simulink model "SC_FFNN_trainlm_15_15_15_15_Dec_8"  (R2021a)
settings: Solver=VariableStepAuto  StartTime=0.0  StopTime=T  FixedStep=0.1  MaxStep=.1  RelTol=1e-3
model workspace (MAT data in the model file):
  T = [0 0.05 0.1 0.15 0.2 0.25 0.3 0.35 0.4 0.45 0.5 0.55 ... (701 elements, 701x1)]
  U = [3.99594136536 3.99594136536 3.99594136536 3.99594136536 3.99594136536 3.99594136536 3.99594136536 3.99594136536 3.99594136536 3.99594136536 3.99594136536 3.99594136536 ... (701 elements, 701x1)]
libraries: neural x66, simulink_extras x2
(part 2 of 3)

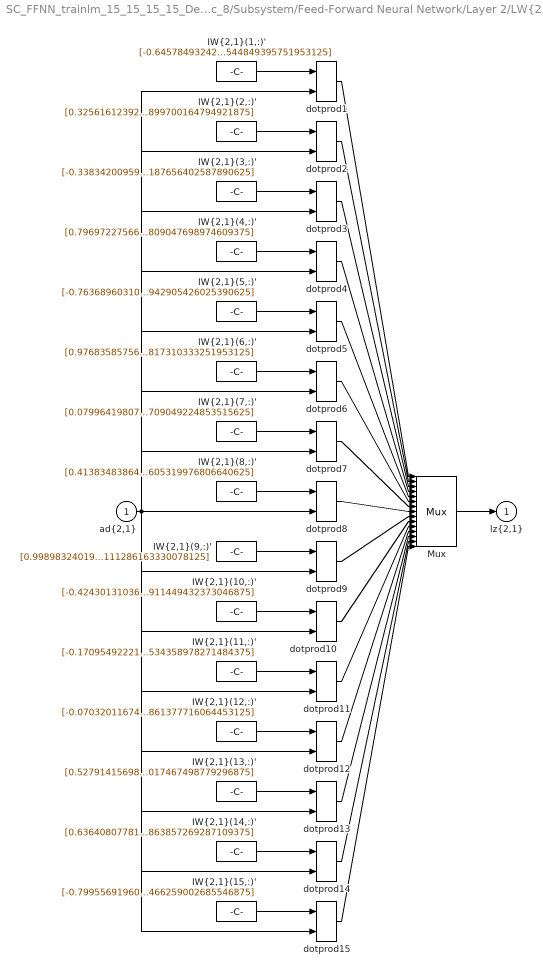
== system SC_FFNN_trainlm_15_15_15_15_Dec_8/Subsystem/Feed-Forward Neural Network/Layer 2/LW{2,1} ==
  "ad{2,1}" : Inport  PortDimensions=15
      mask Display: e = 0.06;c1 = [120 230 180]/255;c2 = ([120 230 180]+0)/(256+128);c3 = ([120 230 180]+128)/(256+128);patch([0 1 1 0],[0 0 1 1],c1);patch([0 1 1 1-e 1-e 0+e],[0 0 1 1-e 0+e 0+e],c2);patch([0 0 1 1-e 0+e 0+e],[0 1 1 1-e 1-e 0+e],c3);plot([0 1 1 0 0],[0 0 1 1 0]);
  "IW{2,1}(1,:)'" : Constant  Value=[-0.6457849324217816988635831876308657228946685791015625;-0.643766092226467190329231016221456229686737060546875;-0.63161180496894697711240951321087777614593505859375;-0.0878846663125170124430951545946300029754638671875;0.0675439035340004156893201070488430559635162353515625;0.3850639727730376105085952076478861272335052490234375;-0.897336227775257899708094555535353720188140869140625;0.4800646559755552544856982422061264514923095703125;-0.5886509570704803184781894742627628147602081298828125;-0.7754320756879466980393544872640632092952728271484375;-0.0247924491321527273868241536547429859638214111328125;-0.81529532256159686909313677460886538028717041015625;-0.367142001707418064171406513196416199207305908203125;0.9758694699049907939070180873386561870574951171875;-0.2984465102282147785928145822254009544849395751953125]
      mask Display: e = 0.06;c1 = [120 150 230]/255;c2 = ([120 150 230]+0)/383;c3 = ([120 150 230]+128)/383;patch([0 1 1 0],[0 0 1 1],c1);patch([0 1 1 1-e 1-e 0+e],[0 0 1 1-e 0+e 0+e],c2);patch([0 0 1 1-e 0+e 0+e],[0 1 1 1-e 1-e 0+e],c3);plot([0 1 1 0 0],[0 0 1 1 0]);disp('weights');
  "IW{2,1}(10,:)'" : Constant  Value=[-0.4243013103697255150592582140234299004077911376953125;-0.0630636001920052979841102569480426609516143798828125;-0.261951995923644875841063139887410216033458709716796875;0.583812871633243357649689642130397260189056396484375;0.2295210394552672783508029397125937975943088531494140625;-0.76428735103558020913538939566933549940586090087890625;-0.553496390046050112943021304090507328510284423828125;0.2202211617163360724003240420643123798072338104248046875;-0.398874395379135215922161705748294480144977569580078125;0.32329322708284891074725919679622165858745574951171875;-0.69601770115887873213722514265100471675395965576171875;-0.76362015015753226254702212827396579086780548095703125;0.8276008215591357242146841599605977535247802734375;0.364025398305722613923052222162368707358837127685546875;-0.1547086935590751277658227991196326911449432373046875]
      mask Display: e = 0.06;c1 = [120 150 230]/255;c2 = ([120 150 230]+0)/383;c3 = ([120 150 230]+128)/383;patch([0 1 1 0],[0 0 1 1],c1);patch([0 1 1 1-e 1-e 0+e],[0 0 1 1-e 0+e 0+e],c2);patch([0 0 1 1-e 0+e 0+e],[0 1 1 1-e 1-e 0+e],c3);plot([0 1 1 0 0],[0 0 1 1 0]);disp('weights');
  "IW{2,1}(11,:)'" : Constant  Value=[-0.170954922213783166995426654466427862644195556640625;0.82426494847924569597807931131683290004730224609375;-0.97343359906549498106187456869520246982574462890625;0.262139998427187048690711890230886638164520263671875;0.0522049315911223832387122456566430628299713134765625;0.0990802140303959077982653980143368244171142578125;0.2814358459318511140878626974881626665592193603515625;0.5787278872838108600973328066174872219562530517578125;-0.5252539605888415508161415345966815948486328125;-0.780489898553896832567033925442956387996673583984375;-0.3683771233222679075680616733734495937824249267578125;-0.8028118145780045455950357791152782738208770751953125;0.4134304353938611509278189259930513799190521240234375;-0.691260389041455258762880475842393934726715087890625;-0.2807873640555287320097477277158759534358978271484375]
      mask Display: e = 0.06;c1 = [120 150 230]/255;c2 = ([120 150 230]+0)/383;c3 = ([120 150 230]+128)/383;patch([0 1 1 0],[0 0 1 1],c1);patch([0 1 1 1-e 1-e 0+e],[0 0 1 1-e 0+e 0+e],c2);patch([0 0 1 1-e 0+e 0+e],[0 1 1 1-e 1-e 0+e],c3);plot([0 1 1 0 0],[0 0 1 1 0]);disp('weights');
  "IW{2,1}(12,:)'" : Constant  Value=[-0.0703201167497253809557378190220333635807037353515625;-0.7919768504412429965810815701843239367008209228515625;0.06419107271674366621549978617622400633990764617919921875;-0.317608463431375775964937702156021259725093841552734375;0.7925487488476712361062936906819231808185577392578125;0.00801786996665575062148700880015894654206931591033935546875;-0.047812738308209347393162857997594983316957950592041015625;0.029586733863963689261655787277049967087805271148681640625;0.345442257577304456805933341456693597137928009033203125;1.329969655156431063147692839265801012516021728515625;1.0607839833820345010195751456194557249546051025390625;-0.3838467293922487311164104539784602820873260498046875;0.1155779335097524285203007821110077202320098876953125;-0.32214951211426579025243199794203974306583404541015625;0.116638399738594245036438223905861377716064453125]
      mask Display: e = 0.06;c1 = [120 150 230]/255;c2 = ([120 150 230]+0)/383;c3 = ([120 150 230]+128)/383;patch([0 1 1 0],[0 0 1 1],c1);patch([0 1 1 1-e 1-e 0+e],[0 0 1 1-e 0+e 0+e],c2);patch([0 0 1 1-e 0+e 0+e],[0 1 1 1-e 1-e 0+e],c3);plot([0 1 1 0 0],[0 0 1 1 0]);disp('weights');
  "IW{2,1}(13,:)'" : Constant  Value=[0.5279141569839131964414491449133493006229400634765625;0.4910921474034346534409678497468121349811553955078125;-0.606683617264736074758957329322583973407745361328125;-0.8382751537393726692926065879873931407928466796875;0.414506970630843074587801311281509697437286376953125;0.7809513583688765248069785229745320975780487060546875;0.3076240451915472906563309152261354029178619384765625;-0.5879442809896107124956188272335566580295562744140625;-0.81700253732117555927061403053812682628631591796875;-0.62507838715662700224129366688430309295654296875;0.3928659780121896982763018968398682773113250732421875;-0.6634974030169444869642347839544527232646942138671875;-0.3731420201268174086095541497343219816684722900390625;-0.6777320563012783072309730414417572319507598876953125;0.4850907314038781503739983236300759017467498779296875]
      mask Display: e = 0.06;c1 = [120 150 230]/255;c2 = ([120 150 230]+0)/383;c3 = ([120 150 230]+128)/383;patch([0 1 1 0],[0 0 1 1],c1);patch([0 1 1 1-e 1-e 0+e],[0 0 1 1-e 0+e 0+e],c2);patch([0 0 1 1-e 0+e 0+e],[0 1 1 1-e 1-e 0+e],c3);plot([0 1 1 0 0],[0 0 1 1 0]);disp('weights');
  "IW{2,1}(14,:)'" : Constant  Value=[0.636408077815341588490127833210863173007965087890625;0.4725349111932770629351807656348682940006256103515625;-0.8132589664898139947268873584107495844364166259765625;0.554481073097886412170964831602759659290313720703125;0.5627541035985543782516060673515312373638153076171875;0.597920557625758686270955877262167632579803466796875;0.498262926207038159276407895958982408046722412109375;-0.8266669052089354874368609671364538371562957763671875;-0.189369160238817446639814079389907419681549072265625;-0.4676423221847223476999033664469607174396514892578125;-0.7493356377816400293312426583725027740001678466796875;-0.6075021554860893235883168017608113586902618408203125;-0.6675928741956986822714270601863972842693328857421875;0.516224862654837135522711832891218364238739013671875;-0.1513304327486186817708357921219430863857269287109375]
      mask Display: e = 0.06;c1 = [120 150 230]/255;c2 = ([120 150 230]+0)/383;c3 = ([120 150 230]+128)/383;patch([0 1 1 0],[0 0 1 1],c1);patch([0 1 1 1-e 1-e 0+e],[0 0 1 1-e 0+e 0+e],c2);patch([0 0 1 1-e 0+e 0+e],[0 1 1 1-e 1-e 0+e],c3);plot([0 1 1 0 0],[0 0 1 1 0]);disp('weights');
  "IW{2,1}(15,:)'" : Constant  Value=[-0.799556919609016869543438588152639567852020263671875;0.12372285056327481100879595032893121242523193359375;-0.3508058136455447506563132265000604093074798583984375;0.982529142477143846434728402527980506420135498046875;-0.2530487716218956517622018509428016841411590576171875;0.44291456538828744005087401092168875038623809814453125;0.499890054502398040181532223868998698890209197998046875;0.56521538701470941390425650752149522304534912109375;-0.71049396982996892990769310927134938538074493408203125;0.44869860757813551099815185807528905570507049560546875;-0.64834895004813952734679105560644529759883880615234375;-0.50962148200618540005990553254378028213977813720703125;0.244994518559790375178408794454298913478851318359375;0.99033985712147754032486091091413982212543487548828125;-0.1412884228475899117682956784847192466259002685546875]
      mask Display: e = 0.06;c1 = [120 150 230]/255;c2 = ([120 150 230]+0)/383;c3 = ([120 150 230]+128)/383;patch([0 1 1 0],[0 0 1 1],c1);patch([0 1 1 1-e 1-e 0+e],[0 0 1 1-e 0+e 0+e],c2);patch([0 0 1 1-e 0+e 0+e],[0 1 1 1-e 1-e 0+e],c3);plot([0 1 1 0 0],[0 0 1 1 0]);disp('weights');
  "IW{2,1}(2,:)'" : Constant  Value=[0.325616123921948830144401654251851141452789306640625;-0.2807301730358393587749787911889143288135528564453125;0.19442270067570976976867314078845083713531494140625;-0.7966612127504897333807321047061122953891754150390625;-0.7816915759150828701962154809734784066677093505859375;0.1133396699280251329611246546846814453601837158203125;-0.854229401802047760838831891305744647979736328125;-0.530346170504191416483763532596640288829803466796875;-0.2234567379043965740237354111741296947002410888671875;0.5688557814878254514923128226655535399913787841796875;0.5379165281177382684774102017399854958057403564453125;-0.9843594128613302185470956828794442117214202880859375;-0.564873381154358700229067835607565939426422119140625;-0.6591359538862333611319854753674007952213287353515625;0.3710714174950744403957969552720896899700164794921875]
      mask Display: e = 0.06;c1 = [120 150 230]/255;c2 = ([120 150 230]+0)/383;c3 = ([120 150 230]+128)/383;patch([0 1 1 0],[0 0 1 1],c1);patch([0 1 1 1-e 1-e 0+e],[0 0 1 1-e 0+e 0+e],c2);patch([0 0 1 1-e 0+e 0+e],[0 1 1 1-e 1-e 0+e],c3);plot([0 1 1 0 0],[0 0 1 1 0]);disp('weights');
  "IW{2,1}(3,:)'" : Constant  Value=[-0.33834200959339089109789711073972284793853759765625;-0.8865906218634176383375233854167163372039794921875;-0.4001260198204221740780894833733327686786651611328125;1.02120211881773759188263284158892929553985595703125;0.70838934016579579999728366601630114018917083740234375;-0.1764984869556638358290001633577048778533935546875;-0.8229450806505591575756852762424387037754058837890625;0.52977589563979499143187013032729737460613250732421875;0.184675824070698435530601955179008655250072479248046875;-0.329453926740678137985440798729541711509227752685546875;-0.1473086768571251481407813344048918224871158599853515625;-0.1490037611855022092743894290833850391209125518798828125;-0.4979163079685278159303152278880588710308074951171875;-0.4844154988559739027920159060158766806125640869140625;-0.4117027324643007801796557032503187656402587890625]
      mask Display: e = 0.06;c1 = [120 150 230]/255;c2 = ([120 150 230]+0)/383;c3 = ([120 150 230]+128)/383;patch([0 1 1 0],[0 0 1 1],c1);patch([0 1 1 1-e 1-e 0+e],[0 0 1 1-e 0+e 0+e],c2);patch([0 0 1 1-e 0+e 0+e],[0 1 1 1-e 1-e 0+e],c3);plot([0 1 1 0 0],[0 0 1 1 0]);disp('weights');
  "IW{2,1}(4,:)'" : Constant  Value=[0.7969722756685990727731905280961655080318450927734375;0.0437713473225584959180878286133520305156707763671875;-0.5997826501763905415742783588939346373081207275390625;-0.253376872142529852016679114967701025307178497314453125;-0.253880698516011638066203204289195127785205841064453125;-0.8411563306374827408973260389757342636585235595703125;0.5967017282279047929449689036118797957897186279296875;0.901428807425623812576986892963759601116180419921875;-0.4921638283901297317157741417759098112583160400390625;0.14982480718348611947732251792331226170063018798828125;-0.48965927940785081151631175089278258383274078369140625;0.300741058062357069502468220889568328857421875;0.785844810571953988898030729615129530429840087890625;-0.2064013627337126788319210390909574925899505615234375;0.0612586077137711182416524025029502809047698974609375]
      mask Display: e = 0.06;c1 = [120 150 230]/255;c2 = ([120 150 230]+0)/383;c3 = ([120 150 230]+128)/383;patch([0 1 1 0],[0 0 1 1],c1);patch([0 1 1 1-e 1-e 0+e],[0 0 1 1-e 0+e 0+e],c2);patch([0 0 1 1-e 0+e 0+e],[0 1 1 1-e 1-e 0+e],c3);plot([0 1 1 0 0],[0 0 1 1 0]);disp('weights');
  "IW{2,1}(5,:)'" : Constant  Value=[-0.763689603106578740465693044825457036495208740234375;-0.3283020506461509224749306667945347726345062255859375;-0.8876177150644160018799766476149670779705047607421875;-0.420784292798006831493040635905344970524311065673828125;-0.25756149257502658489471514258184470236301422119140625;0.5461900791356344431193292621173895895481109619140625;0.759983566893656092844366867211647331714630126953125;0.89502295944068255284520319037255831062793731689453125;0.20025355222368601548765809639007784426212310791015625;1.16417871898486691151219929452054202556610107421875;-0.69985601393419327731493240207782946527004241943359375;0.48398892509027202635252251639030873775482177734375;0.406446449112582097740187236922793090343475341796875;-0.8919620843481268490648972147027961909770965576171875;0.6648467725703677277948600021773017942905426025390625]
      mask Display: e = 0.06;c1 = [120 150 230]/255;c2 = ([120 150 230]+0)/383;c3 = ([120 150 230]+128)/383;patch([0 1 1 0],[0 0 1 1],c1);patch([0 1 1 1-e 1-e 0+e],[0 0 1 1-e 0+e 0+e],c2);patch([0 0 1 1-e 0+e 0+e],[0 1 1 1-e 1-e 0+e],c3);plot([0 1 1 0 0],[0 0 1 1 0]);disp('weights');
  "IW{2,1}(6,:)'" : Constant  Value=[0.9768358575699611634490793221630156040191650390625;-0.6486619406486784367160680631059221923351287841796875;0.958483109691663504037251186673529446125030517578125;-0.7977771644401168149585146238678134977817535400390625;0.71947601476091549432823057941277511417865753173828125;-0.1375190134754562254482124217247474007308483123779296875;0.399138242939769793959925436865887604653835296630859375;-0.635155129528707451669333750032819807529449462890625;-0.0310392552036391489167499457835219800472259521484375;-0.14794002574780462655468227239907719194889068603515625;0.5082928105306112609440560845541767776012420654296875;-0.371918306418970001647750223128241486847400665283203125;0.1114758854387731812352058113901875913143157958984375;0.8305364916151283249945436182315461337566375732421875;0.1949803837451586918660950686899013817310333251953125]
      mask Display: e = 0.06;c1 = [120 150 230]/255;c2 = ([120 150 230]+0)/383;c3 = ([120 150 230]+128)/383;patch([0 1 1 0],[0 0 1 1],c1);patch([0 1 1 1-e 1-e 0+e],[0 0 1 1-e 0+e 0+e],c2);patch([0 0 1 1-e 0+e 0+e],[0 1 1 1-e 1-e 0+e],c3);plot([0 1 1 0 0],[0 0 1 1 0]);disp('weights');
  "IW{2,1}(7,:)'" : Constant  Value=[0.0799641980758583059696320560760796070098876953125;-0.582106652013729242156614418490789830684661865234375;-0.62139260847947508370481273232144303619861602783203125;-0.4272172387787180891649541081278584897518157958984375;-0.987011545743446294665091045317240059375762939453125;0.215731814525891518741218533250503242015838623046875;-0.7366046234336669495945670860237441956996917724609375;-0.36860428836198388946598925031139515340328216552734375;-0.6963089497674668226778749158256687223911285400390625;0.27212084372591183178968776701367460191249847412109375;-0.2763829701371836033985118774580769240856170654296875;-0.7166785917443989628594636087655089795589447021484375;-0.631132664484693517437108312151394784450531005859375;-0.1944020438064752998030826347530819475650787353515625;-0.3293773385895077954188536750734783709049224853515625]
      mask Display: e = 0.06;c1 = [120 150 230]/255;c2 = ([120 150 230]+0)/383;c3 = ([120 150 230]+128)/383;patch([0 1 1 0],[0 0 1 1],c1);patch([0 1 1 1-e 1-e 0+e],[0 0 1 1-e 0+e 0+e],c2);patch([0 0 1 1-e 0+e 0+e],[0 1 1 1-e 1-e 0+e],c3);plot([0 1 1 0 0],[0 0 1 1 0]);disp('weights');
  "IW{2,1}(8,:)'" : Constant  Value=[0.413834838645525504574607111862860620021820068359375;0.8103071180089280733938039702479727566242218017578125;-0.43990784105602587228389666051953099668025970458984375;-0.70097915133558508227196170992101542651653289794921875;-0.78846063140701172500257598585449159145355224609375;0.463939307580775894823688076940015889704227447509765625;0.250627654122016263471550701069645583629608154296875;-0.4437061320009487719318030940485186874866485595703125;0.58837738063915445696494543881271965801715850830078125;0.3073992544338908228240825337707065045833587646484375;-0.296062152743406914456869571949937380850315093994140625;0.257003612065806297248826695067691616714000701904296875;-0.5759383149353585196195126627571880817413330078125;0.72878493283118606083093027336872182786464691162109375;-0.401549953333786735498733833082951605319976806640625]
      mask Display: e = 0.06;c1 = [120 150 230]/255;c2 = ([120 150 230]+0)/383;c3 = ([120 150 230]+128)/383;patch([0 1 1 0],[0 0 1 1],c1);patch([0 1 1 1-e 1-e 0+e],[0 0 1 1-e 0+e 0+e],c2);patch([0 0 1 1-e 0+e 0+e],[0 1 1 1-e 1-e 0+e],c3);plot([0 1 1 0 0],[0 0 1 1 0]);disp('weights');
  "IW{2,1}(9,:)'" : Constant  Value=[0.9989832401954092944151852861978113651275634765625;0.35078235467249374579523646389134228229522705078125;-0.892491215582572383624437861726619303226470947265625;0.010856284915405911561947505106218159198760986328125;0.3358322431472473557079183592577464878559112548828125;-0.7903735160530007686219278184580616652965545654296875;-0.7792930387153027549373973670299164950847625732421875;0.3700569453232185335167514494969509541988372802734375;-0.7987873552751569850016721829888410866260528564453125;-0.1347153477057989601206600127625279128551483154296875;0.2197143385804321003007544277352280914783477783203125;-0.7470002693413941852185189418378286063671112060546875;-0.8453063837746463971001276149763725697994232177734375;-0.195632029555030673151350129046477377414703369140625;-0.0948149168613519055526239753817208111286163330078125]
      mask Display: e = 0.06;c1 = [120 150 230]/255;c2 = ([120 150 230]+0)/383;c3 = ([120 150 230]+128)/383;patch([0 1 1 0],[0 0 1 1],c1);patch([0 1 1 1-e 1-e 0+e],[0 0 1 1-e 0+e 0+e],c2);patch([0 0 1 1-e 0+e 0+e],[0 1 1 1-e 1-e 0+e],c3);plot([0 1 1 0 0],[0 0 1 1 0]);disp('weights');
  Mux : Mux  Inputs=15
      mask Display: e = 0.06;c1 = [120 150 230]/255;c2 = ([120 150 230]+0)/383;c3 = ([120 150 230]+128)/383;patch([0 1 1 0],[0 0 1 1],c1);patch([0 1 1 1-e 1-e 0+e],[0 0 1 1-e 0+e 0+e],c2);patch([0 0 1 1-e 0+e 0+e],[0 1 1 1-e 1-e 0+e],c3);plot([0 1 1 0 0],[0 0 1 1 0]);disp('Mux');
  dotprod{1..15} (15 alike) : neural/Weight Functions/dotprod
  "lz{2,1}" : Outport
      mask Display: e = 0.06;c1 = [120 230 180]/255;c2 = ([120 230 180]+0)/(256+128);c3 = ([120 230 180]+128)/(256+128);patch([0 1 1 0],[0 0 1 1],c1);patch([0 1 1 1-e 1-e 0+e],[0 0 1 1-e 0+e 0+e],c2);patch([0 0 1 1-e 0+e 0+e],[0 1 1 1-e 1-e 0+e],c3);plot([0 1 1 0 0],[0 0 1 1 0]);
  wires:
  "IW{2,1}(1,:)'"/1 -> dotprod1/1
  "ad{2,1}"/1 -> dotprod1/2, dotprod2/2, dotprod3/2, dotprod4/2, dotprod5/2, dotprod6/2, dotprod7/2, dotprod8/2, dotprod9/2, dotprod10/2, dotprod11/2, dotprod12/2, dotprod13/2, dotprod14/2, dotprod15/2
  dotprod1/1 -> Mux/1
  "IW{2,1}(2,:)'"/1 -> dotprod2/1
  dotprod2/1 -> Mux/2
  "IW{2,1}(3,:)'"/1 -> dotprod3/1
  dotprod3/1 -> Mux/3
  "IW{2,1}(4,:)'"/1 -> dotprod4/1
  dotprod4/1 -> Mux/4
  "IW{2,1}(5,:)'"/1 -> dotprod5/1
  dotprod5/1 -> Mux/5
  "IW{2,1}(6,:)'"/1 -> dotprod6/1
  dotprod6/1 -> Mux/6
  "IW{2,1}(7,:)'"/1 -> dotprod7/1
  dotprod7/1 -> Mux/7
  "IW{2,1}(8,:)'"/1 -> dotprod8/1
  dotprod8/1 -> Mux/8
  "IW{2,1}(9,:)'"/1 -> dotprod9/1
  dotprod9/1 -> Mux/9
  "IW{2,1}(10,:)'"/1 -> dotprod10/1
  dotprod10/1 -> Mux/10
  "IW{2,1}(11,:)'"/1 -> dotprod11/1
  dotprod11/1 -> Mux/11
  "IW{2,1}(12,:)'"/1 -> dotprod12/1
  dotprod12/1 -> Mux/12
  "IW{2,1}(13,:)'"/1 -> dotprod13/1
  dotprod13/1 -> Mux/13
  "IW{2,1}(14,:)'"/1 -> dotprod14/1
  dotprod14/1 -> Mux/14
  "IW{2,1}(15,:)'"/1 -> dotprod15/1
  dotprod15/1 -> Mux/15
  Mux/1 -> "lz{2,1}"/1

== system SC_FFNN_trainlm_15_15_15_15_Dec_8/Subsystem/Feed-Forward Neural Network/Layer 3/Delays 1 ==
  "p{3}" : Inport  PortDimensions=15
      mask Display: e = 0.06;c1 = [120 230 180]/255;c2 = ([120 230 180]+0)/(256+128);c3 = ([120 230 180]+128)/(256+128);patch([0 1 1 0],[0 0 1 1],c1);patch([0 1 1 1-e 1-e 0+e],[0 0 1 1-e 0+e 0+e],c2);patch([0 0 1 1-e 0+e 0+e],[0 1 1 1-e 1-e 0+e],c3);plot([0 1 1 0 0],[0 0 1 1 0]);
  mux : Mux  Inputs=1
      mask Display: e = 0.06;c1 = [120 150 230]/255;c2 = ([120 150 230]+0)/383;c3 = ([120 150 230]+128)/383;patch([0 1 1 0],[0 0 1 1],c1);patch([0 1 1 1-e 1-e 0+e],[0 0 1 1-e 0+e 0+e],c2);patch([0 0 1 1-e 0+e 0+e],[0 1 1 1-e 1-e 0+e],c3);plot([0 1 1 0 0],[0 0 1 1 0]);disp('Mux')
  "pd{3,2}" : Outport
      mask Display: e = 0.06;c1 = [120 230 180]/255;c2 = ([120 230 180]+0)/(256+128);c3 = ([120 230 180]+128)/(256+128);patch([0 1 1 0],[0 0 1 1],c1);patch([0 1 1 1-e 1-e 0+e],[0 0 1 1-e 0+e 0+e],c2);patch([0 0 1 1-e 0+e 0+e],[0 1 1 1-e 1-e 0+e],c3);plot([0 1 1 0 0],[0 0 1 1 0]);
  wires:
  "p{3}"/1 -> mux/1
  mux/1 -> "pd{3,2}"/1

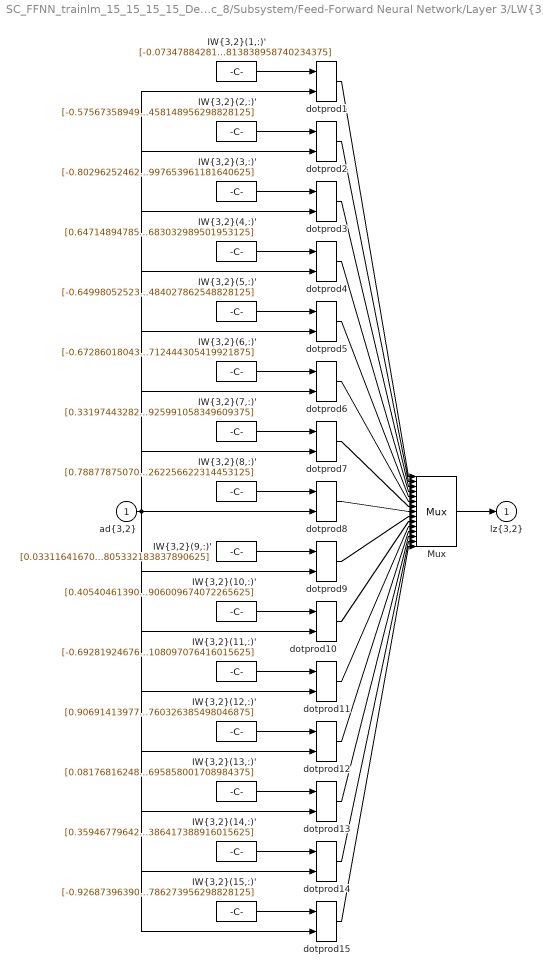
== system SC_FFNN_trainlm_15_15_15_15_Dec_8/Subsystem/Feed-Forward Neural Network/Layer 3/LW{3,2} ==
  "ad{3,2}" : Inport  PortDimensions=15
      mask Display: e = 0.06;c1 = [120 230 180]/255;c2 = ([120 230 180]+0)/(256+128);c3 = ([120 230 180]+128)/(256+128);patch([0 1 1 0],[0 0 1 1],c1);patch([0 1 1 1-e 1-e 0+e],[0 0 1 1-e 0+e 0+e],c2);patch([0 0 1 1-e 0+e 0+e],[0 1 1 1-e 1-e 0+e],c3);plot([0 1 1 0 0],[0 0 1 1 0]);
  "IW{3,2}(1,:)'" : Constant  Value=[-0.07347884281256167327001094236038625240325927734375;0.61840770258758670507859278586693108081817626953125;0.8005017582493969552359658337081782519817352294921875;-0.2544500328198180394423388861468993127346038818359375;0.275233375677362890332489087086287327110767364501953125;-0.51656601115191314033125991045380942523479461669921875;0.6262256272215214192300436479854397475719451904296875;1.0352167510154359764129594623227603733539581298828125;0.2328869701713702777823300493764691054821014404296875;-0.17681297318493083281509825610555708408355712890625;-0.17314542195836946092413199949078261852264404296875;-0.427514788049068894526527628840995021164417266845703125;0.7917831475851364597673409662093035876750946044921875;0.002565826406430549155857079313136637210845947265625;0.46493747286896702775038647814653813838958740234375]
      mask Display: e = 0.06;c1 = [120 150 230]/255;c2 = ([120 150 230]+0)/383;c3 = ([120 150 230]+128)/383;patch([0 1 1 0],[0 0 1 1],c1);patch([0 1 1 1-e 1-e 0+e],[0 0 1 1-e 0+e 0+e],c2);patch([0 0 1 1-e 0+e 0+e],[0 1 1 1-e 1-e 0+e],c3);plot([0 1 1 0 0],[0 0 1 1 0]);disp('weights');
  "IW{3,2}(10,:)'" : Constant  Value=[0.4054046139009506166672736071632243692874908447265625;-0.489226519023898465121646950137801468372344970703125;0.16188259861384646232096429230296052992343902587890625;0.76905186575705120066714925997075624763965606689453125;0.72275122526789281618420091035659424960613250732421875;-0.279153237437250900665475228379364125430583953857421875;0.445048886645755426005877097850316204130649566650390625;-0.006568886540310924816721271923825042904354631900787353515625;-0.3266014712170477451991246198303997516632080078125;0.608827311640479873489084639004431664943695068359375;0.8446639955925514531287490171962417662143707275390625;1.0766719361305125968186757745570503175258636474609375;0.0203050395305004460766440388397313654422760009765625;0.8349876648322338557051125462749041616916656494140625;0.451233825686171263757984206677065230906009674072265625]
      mask Display: e = 0.06;c1 = [120 150 230]/255;c2 = ([120 150 230]+0)/383;c3 = ([120 150 230]+128)/383;patch([0 1 1 0],[0 0 1 1],c1);patch([0 1 1 1-e 1-e 0+e],[0 0 1 1-e 0+e 0+e],c2);patch([0 0 1 1-e 0+e 0+e],[0 1 1 1-e 1-e 0+e],c3);plot([0 1 1 0 0],[0 0 1 1 0]);disp('weights');
  "IW{3,2}(11,:)'" : Constant  Value=[-0.692819246761199547535170495393685996532440185546875;-0.9589284506836308619170949896215461194515228271484375;0.430425029571680273221545576234348118305206298828125;0.26237746853802246249642848852090537548065185546875;0.1410184172399946145315396961450460366904735565185546875;0.45441163057096323196759612983441911637783050537109375;0.9722084837919402477979247123585082590579986572265625;-0.72408495328459310247382063607801683247089385986328125;0.3247637207989624297255204510292969644069671630859375;-0.290931390086156316243659603060223162174224853515625;0.5419084413478489903326362764346413314342498779296875;-0.7715724845926617003755154655664227902889251708984375;0.812728646530429532646166990161873400211334228515625;0.4271480231886315426237388237495906651020050048828125;-0.34088090365741463561022328576655127108097076416015625]
      mask Display: e = 0.06;c1 = [120 150 230]/255;c2 = ([120 150 230]+0)/383;c3 = ([120 150 230]+128)/383;patch([0 1 1 0],[0 0 1 1],c1);patch([0 1 1 1-e 1-e 0+e],[0 0 1 1-e 0+e 0+e],c2);patch([0 0 1 1-e 0+e 0+e],[0 1 1 1-e 1-e 0+e],c3);plot([0 1 1 0 0],[0 0 1 1 0]);disp('weights');
  "IW{3,2}(12,:)'" : Constant  Value=[0.90691413977249535349756115465424954891204833984375;0.8473512252408144096449404969462193548679351806640625;0.284121656867704519555672959540970623493194580078125;-0.2898526962423020325587685874779708683490753173828125;-0.646289884749394527574395397095941007137298583984375;-0.9567003707393870737263341652578674256801605224609375;-0.940016099461220111521697617718018591403961181640625;-0.5643968125757508058626399360946379601955413818359375;-0.511669426419441464304327382706105709075927734375;0.9425176303668114652367648886865936219692230224609375;-0.9146802881299025411721004275023005902767181396484375;-0.6355449887978885659123307050322182476520538330078125;0.2578478773046357641618442357867024838924407958984375;0.2366747672438800353944543530815280973911285400390625;0.238943110355559706903250116738490760326385498046875]
      mask Display: e = 0.06;c1 = [120 150 230]/255;c2 = ([120 150 230]+0)/383;c3 = ([120 150 230]+128)/383;patch([0 1 1 0],[0 0 1 1],c1);patch([0 1 1 1-e 1-e 0+e],[0 0 1 1-e 0+e 0+e],c2);patch([0 0 1 1-e 0+e 0+e],[0 1 1 1-e 1-e 0+e],c3);plot([0 1 1 0 0],[0 0 1 1 0]);disp('weights');
  "IW{3,2}(13,:)'" : Constant  Value=[0.0817681624829529329900879019987769424915313720703125;0.3073997780165058646417719501187093555927276611328125;-0.2516989390348756128190643721609376370906829833984375;0.88896374341652728556795182157657109200954437255859375;0.87507300512998498209782383128185756504535675048828125;0.856851354818488619713434673030860722064971923828125;0.1976529382039062532339102062906022183597087860107421875;-0.50149677627274680258295802559587173163890838623046875;-0.408985498336806418961941744782961905002593994140625;-0.06610286600487262631542506596815655939280986785888671875;-0.243627725899562275202470118529163300991058349609375;-0.5024038075255317092882023644051514565944671630859375;-0.7969322223753756428976657844032160937786102294921875;-0.313424219517309143867578313802368938922882080078125;-0.447503776689701648905383990495465695858001708984375]
      mask Display: e = 0.06;c1 = [120 150 230]/255;c2 = ([120 150 230]+0)/383;c3 = ([120 150 230]+128)/383;patch([0 1 1 0],[0 0 1 1],c1);patch([0 1 1 1-e 1-e 0+e],[0 0 1 1-e 0+e 0+e],c2);patch([0 0 1 1-e 0+e 0+e],[0 1 1 1-e 1-e 0+e],c3);plot([0 1 1 0 0],[0 0 1 1 0]);disp('weights');
  "IW{3,2}(14,:)'" : Constant  Value=[0.3594677964209338494327994339982978999614715576171875;0.8652271440971281979415152818546630442142486572265625;-0.2130306621080632345499594748616800643503665924072265625;-0.476954499087445416005692777616786770522594451904296875;-0.3318848384136205975636357834446243941783905029296875;0.75004804428943006033847495928057469427585601806640625;-0.75887602265938569612302444511442445218563079833984375;-0.8083676326311881599195885428343899548053741455078125;0.360356742461004131428126129321753978729248046875;0.9457401044200761663915955068659968674182891845703125;0.4086792489667352423765578350867144763469696044921875;0.1046673122844769820982691044264356605708599090576171875;-0.21829049454729076984449420706368982791900634765625;0.8720546533795394683608037666999734938144683837890625;0.540739063778151063388577313162386417388916015625]
      mask Display: e = 0.06;c1 = [120 150 230]/255;c2 = ([120 150 230]+0)/383;c3 = ([120 150 230]+128)/383;patch([0 1 1 0],[0 0 1 1],c1);patch([0 1 1 1-e 1-e 0+e],[0 0 1 1-e 0+e 0+e],c2);patch([0 0 1 1-e 0+e 0+e],[0 1 1 1-e 1-e 0+e],c3);plot([0 1 1 0 0],[0 0 1 1 0]);disp('weights');
  "IW{3,2}(15,:)'" : Constant  Value=[-0.926873963903094288951933776843361556529998779296875;-0.6729752629449488043889004984521307051181793212890625;0.61327854839882156579022876030649058520793914794921875;0.414994028783071067234544671009643934667110443115234375;0.71420625952947036640949818320223130285739898681640625;0.62815896838087159625985123057034797966480255126953125;0.64231420971789365825799222875502891838550567626953125;-0.63447623985525181122824278645566664636135101318359375;0.0556936608375957487027108072652481496334075927734375;0.042453133165891672462510797458890010602772235870361328125;0.4590260910092938129167805527686141431331634521484375;-0.6776587744283866232564150777761824429035186767578125;-0.89076676955268485613714801729656755924224853515625;-0.7504519186790148399524014166672714054584503173828125;-0.098386456268748034847959615945001132786273956298828125]
      mask Display: e = 0.06;c1 = [120 150 230]/255;c2 = ([120 150 230]+0)/383;c3 = ([120 150 230]+128)/383;patch([0 1 1 0],[0 0 1 1],c1);patch([0 1 1 1-e 1-e 0+e],[0 0 1 1-e 0+e 0+e],c2);patch([0 0 1 1-e 0+e 0+e],[0 1 1 1-e 1-e 0+e],c3);plot([0 1 1 0 0],[0 0 1 1 0]);disp('weights');
  "IW{3,2}(2,:)'" : Constant  Value=[-0.5756735894901312544646998503594659268856048583984375;0.4972377435523942512674011595663614571094512939453125;0.589315770777506298117032201844267547130584716796875;0.6290795458013025420740405024844221770763397216796875;-0.2255091370337301004411756366607733070850372314453125;-0.2528723847147100745047509917640127241611480712890625;-0.23338736274894156252912580384872853755950927734375;-0.8661074832044997062752145211561582982540130615234375;0.8793220203221334685395049746148288249969482421875;0.20527643607279433268786306143738329410552978515625;-0.5645358632853991753819400400971062481403350830078125;-0.4618905364532699397983606104389764368534088134765625;-0.801820700636370897740334839909337460994720458984375;-0.1365576562315056197149942818214185535907745361328125;0.29295486485162758327760457177646458148956298828125]
      mask Display: e = 0.06;c1 = [120 150 230]/255;c2 = ([120 150 230]+0)/383;c3 = ([120 150 230]+128)/383;patch([0 1 1 0],[0 0 1 1],c1);patch([0 1 1 1-e 1-e 0+e],[0 0 1 1-e 0+e 0+e],c2);patch([0 0 1 1-e 0+e 0+e],[0 1 1 1-e 1-e 0+e],c3);plot([0 1 1 0 0],[0 0 1 1 0]);disp('weights');
  "IW{3,2}(3,:)'" : Constant  Value=[-0.8029625246237832580931126358336769044399261474609375;-0.7596259640258387069167156369076110422611236572265625;0.07279440332663351942432683472361532039940357208251953125;0.314083181970030322904818831375450827181339263916015625;-0.89384215988824700094284025908564217388629913330078125;-0.59377545863063285747074360187980346381664276123046875;0.1692646999590492196130497859485330991446971893310546875;0.56253113840821489244348185820854268968105316162109375;-0.291088538065342294913762088981457054615020751953125;0.434267472054608305587208860742975957691669464111328125;-0.748690825274747506767880622646771371364593505859375;0.430858274071968805341015240628621540963649749755859375;-0.9116688564746777689862256011110730469226837158203125;0.9951206990243781635996356271789409220218658447265625;0.60759303411711018672036743737407959997653961181640625]
      mask Display: e = 0.06;c1 = [120 150 230]/255;c2 = ([120 150 230]+0)/383;c3 = ([120 150 230]+128)/383;patch([0 1 1 0],[0 0 1 1],c1);patch([0 1 1 1-e 1-e 0+e],[0 0 1 1-e 0+e 0+e],c2);patch([0 0 1 1-e 0+e 0+e],[0 1 1 1-e 1-e 0+e],c3);plot([0 1 1 0 0],[0 0 1 1 0]);disp('weights');
  "IW{3,2}(4,:)'" : Constant  Value=[0.64714894785567711466001128428615629673004150390625;0.0500903295252175251306425707298330962657928466796875;-0.1199288084794927211618187357089482247829437255859375;0.7045277806876912851663519177236594259738922119140625;-0.9354813119764047169013565508066676557064056396484375;0.328022716264994074197858253683079965412616729736328125;0.1509897194056277758278383771539665758609771728515625;-0.9071015483007915936042309112963266670703887939453125;-0.178741819880972041545419415342621505260467529296875;0.1670663485239172185714551233104430139064788818359375;-0.3821708128663694470361633648280985653400421142578125;-0.2040287909842075364519331515111844055354595184326171875;0.1145903116095237095350967138074338436126708984375;0.623205161990645795100363102392293512821197509765625;-0.1273395741548444537460937908690539188683032989501953125]
      mask Display: e = 0.06;c1 = [120 150 230]/255;c2 = ([120 150 230]+0)/383;c3 = ([120 150 230]+128)/383;patch([0 1 1 0],[0 0 1 1],c1);patch([0 1 1 1-e 1-e 0+e],[0 0 1 1-e 0+e 0+e],c2);patch([0 0 1 1-e 0+e 0+e],[0 1 1 1-e 1-e 0+e],c3);plot([0 1 1 0 0],[0 0 1 1 0]);disp('weights');
  "IW{3,2}(5,:)'" : Constant  Value=[-0.64998052523584082251772997551597654819488525390625;-0.3483327424735016553114519410883076488971710205078125;-0.5551892738572643537509065936319530010223388671875;0.0159070552395294724512542217098598484881222248077392578125;-0.291628649818918728175987098438781686127185821533203125;-0.3949767246108120133385455119423568248748779296875;0.1046868059475021539572736628542770631611347198486328125;0.45653332926602396835136232766672037541866302490234375;0.968698833968903105784420404233969748020172119140625;0.252986660918413763798895388390519656240940093994140625;0.4522088633296637016911745377001352608203887939453125;0.13802087878038216128828707951470278203487396240234375;0.54499013437524812530909912311471998691558837890625;-0.0286966602039646634381142575875855982303619384765625;0.404407297391073783376924666299601085484027862548828125]
      mask Display: e = 0.06;c1 = [120 150 230]/255;c2 = ([120 150 230]+0)/383;c3 = ([120 150 230]+128)/383;patch([0 1 1 0],[0 0 1 1],c1);patch([0 1 1 1-e 1-e 0+e],[0 0 1 1-e 0+e 0+e],c2);patch([0 0 1 1-e 0+e 0+e],[0 1 1 1-e 1-e 0+e],c3);plot([0 1 1 0 0],[0 0 1 1 0]);disp('weights');
  "IW{3,2}(6,:)'" : Constant  Value=[-0.672860180430013610219930342282168567180633544921875;0.0928988798061369802638864712207578122615814208984375;0.5038927877348999828654996235854923725128173828125;0.271322777722753816220802036696113646030426025390625;-0.6317994211449775576738829840905964374542236328125;-0.909897785052851570952725523966364562511444091796875;-0.44986048835612990615118178538978099822998046875;0.5674729601664372236058397902525030076503753662109375;0.8911583780705252255671666716807521879673004150390625;0.1671412375154288643130939817638136446475982666015625;0.565744145958246402727809254429303109645843505859375;-0.52711013471817924624929219135083258152008056640625;-0.3761198850074622956896064351894892752170562744140625;0.7888955111347863979887051755213178694248199462890625;0.6704410209562610134526039473712444305419921875]
      mask Display: e = 0.06;c1 = [120 150 230]/255;c2 = ([120 150 230]+0)/383;c3 = ([120 150 230]+128)/383;patch([0 1 1 0],[0 0 1 1],c1);patch([0 1 1 1-e 1-e 0+e],[0 0 1 1-e 0+e 0+e],c2);patch([0 0 1 1-e 0+e 0+e],[0 1 1 1-e 1-e 0+e],c3);plot([0 1 1 0 0],[0 0 1 1 0]);disp('weights');
  "IW{3,2}(7,:)'" : Constant  Value=[0.3319744328222211660062157534412108361721038818359375;-0.20223849523360204472055556834675371646881103515625;-0.535260506952312198336585424840450286865234375;0.9800193831792254339774217442027293145656585693359375;0.6496406649583692516358723878511227667331695556640625;0.6077079965938481098675083558191545307636260986328125;-0.51782128171345209732834291571634821593761444091796875;0.29824973779517127692173517061746679246425628662109375;0.3532893568670782968865751172415912151336669921875;-0.01927110067193148201791785822933888994157314300537109375;0.3875752299737944550628299111849628388881683349609375;-0.84653279923863966605068753779050894081592559814453125;-0.642035041371329828763236946542747318744659423828125;-0.7249068104658704658760370875825174152851104736328125;0.06193245348217890633435445124632678925991058349609375]
      mask Display: e = 0.06;c1 = [120 150 230]/255;c2 = ([120 150 230]+0)/383;c3 = ([120 150 230]+128)/383;patch([0 1 1 0],[0 0 1 1],c1);patch([0 1 1 1-e 1-e 0+e],[0 0 1 1-e 0+e 0+e],c2);patch([0 0 1 1-e 0+e 0+e],[0 1 1 1-e 1-e 0+e],c3);plot([0 1 1 0 0],[0 0 1 1 0]);disp('weights');
  "IW{3,2}(8,:)'" : Constant  Value=[0.7887787507084855764816211376455612480640411376953125;-0.16981322677390675579545131768099963665008544921875;-1.0864004786316134865131743936217390000820159912109375;-0.2424286362113993453792915033773169852793216705322265625;-0.434353102284060155202638497939915396273136138916015625;-0.12684184097254813661237449196050874888896942138671875;-0.09970884849092097323985939283375046215951442718505859375;0.65510554240750540344606633880175650119781494140625;0.97660452462657243444255072972737252712249755859375;-0.88619842245435587191337845069938339293003082275390625;-0.98039549547387583317004100535996258258819580078125;0.6483045214846339110437156705302186310291290283203125;-0.3220886435045635654006446202402003109455108642578125;-0.2199901711094292000581162938033230602741241455078125;-0.037319838806250123230956461384266731329262256622314453125]
      mask Display: e = 0.06;c1 = [120 150 230]/255;c2 = ([120 150 230]+0)/383;c3 = ([120 150 230]+128)/383;patch([0 1 1 0],[0 0 1 1],c1);patch([0 1 1 1-e 1-e 0+e],[0 0 1 1-e 0+e 0+e],c2);patch([0 0 1 1-e 0+e 0+e],[0 1 1 1-e 1-e 0+e],c3);plot([0 1 1 0 0],[0 0 1 1 0]);disp('weights');
  "IW{3,2}(9,:)'" : Constant  Value=[0.0331164167025408406885844669886864721775054931640625;-0.63852447949041124530822344240732491016387939453125;0.420413397206550409901382181487861089408397674560546875;-0.79477789450197822151977788962540216743946075439453125;0.69748447462870000190804375961306504905223846435546875;0.71375481446864863510626264542224816977977752685546875;-0.589991171846909079334864145494066178798675537109375;0.808507214881688529573011692264117300510406494140625;0.5336627744331885470074894328718073666095733642578125;0.4186038649462167082759833647287450730800628662109375;0.686426676021019144258161759353242814540863037109375;0.376268842643249279422690278806840069591999053955078125;-0.5797087259128959058074315180419944226741790771484375;0.854712449996249734596176494960673153400421142578125;1.1900732800081395001967621283256448805332183837890625]
      mask Display: e = 0.06;c1 = [120 150 230]/255;c2 = ([120 150 230]+0)/383;c3 = ([120 150 230]+128)/383;patch([0 1 1 0],[0 0 1 1],c1);patch([0 1 1 1-e 1-e 0+e],[0 0 1 1-e 0+e 0+e],c2);patch([0 0 1 1-e 0+e 0+e],[0 1 1 1-e 1-e 0+e],c3);plot([0 1 1 0 0],[0 0 1 1 0]);disp('weights');
  Mux : Mux  Inputs=15
      mask Display: e = 0.06;c1 = [120 150 230]/255;c2 = ([120 150 230]+0)/383;c3 = ([120 150 230]+128)/383;patch([0 1 1 0],[0 0 1 1],c1);patch([0 1 1 1-e 1-e 0+e],[0 0 1 1-e 0+e 0+e],c2);patch([0 0 1 1-e 0+e 0+e],[0 1 1 1-e 1-e 0+e],c3);plot([0 1 1 0 0],[0 0 1 1 0]);disp('Mux');
  dotprod{1..15} (15 alike) : neural/Weight Functions/dotprod
  "lz{3,2}" : Outport
      mask Display: e = 0.06;c1 = [120 230 180]/255;c2 = ([120 230 180]+0)/(256+128);c3 = ([120 230 180]+128)/(256+128);patch([0 1 1 0],[0 0 1 1],c1);patch([0 1 1 1-e 1-e 0+e],[0 0 1 1-e 0+e 0+e],c2);patch([0 0 1 1-e 0+e 0+e],[0 1 1 1-e 1-e 0+e],c3);plot([0 1 1 0 0],[0 0 1 1 0]);
  wires:
  "IW{3,2}(1,:)'"/1 -> dotprod1/1
  "ad{3,2}"/1 -> dotprod1/2, dotprod2/2, dotprod3/2, dotprod4/2, dotprod5/2, dotprod6/2, dotprod7/2, dotprod8/2, dotprod9/2, dotprod10/2, dotprod11/2, dotprod12/2, dotprod13/2, dotprod14/2, dotprod15/2
  dotprod1/1 -> Mux/1
  "IW{3,2}(2,:)'"/1 -> dotprod2/1
  dotprod2/1 -> Mux/2
  "IW{3,2}(3,:)'"/1 -> dotprod3/1
  dotprod3/1 -> Mux/3
  "IW{3,2}(4,:)'"/1 -> dotprod4/1
  dotprod4/1 -> Mux/4
  "IW{3,2}(5,:)'"/1 -> dotprod5/1
  dotprod5/1 -> Mux/5
  "IW{3,2}(6,:)'"/1 -> dotprod6/1
  dotprod6/1 -> Mux/6
  "IW{3,2}(7,:)'"/1 -> dotprod7/1
  dotprod7/1 -> Mux/7
  "IW{3,2}(8,:)'"/1 -> dotprod8/1
  dotprod8/1 -> Mux/8
  "IW{3,2}(9,:)'"/1 -> dotprod9/1
  dotprod9/1 -> Mux/9
  "IW{3,2}(10,:)'"/1 -> dotprod10/1
  dotprod10/1 -> Mux/10
  "IW{3,2}(11,:)'"/1 -> dotprod11/1
  dotprod11/1 -> Mux/11
  "IW{3,2}(12,:)'"/1 -> dotprod12/1
  dotprod12/1 -> Mux/12
  "IW{3,2}(13,:)'"/1 -> dotprod13/1
  dotprod13/1 -> Mux/13
  "IW{3,2}(14,:)'"/1 -> dotprod14/1
  dotprod14/1 -> Mux/14
  "IW{3,2}(15,:)'"/1 -> dotprod15/1
  dotprod15/1 -> Mux/15
  Mux/1 -> "lz{3,2}"/1

== system SC_FFNN_trainlm_15_15_15_15_Dec_8/Subsystem/Feed-Forward Neural Network/Layer 4/Delays 1 ==
  "p{4}" : Inport  PortDimensions=15
      mask Display: e = 0.06;c1 = [120 230 180]/255;c2 = ([120 230 180]+0)/(256+128);c3 = ([120 230 180]+128)/(256+128);patch([0 1 1 0],[0 0 1 1],c1);patch([0 1 1 1-e 1-e 0+e],[0 0 1 1-e 0+e 0+e],c2);patch([0 0 1 1-e 0+e 0+e],[0 1 1 1-e 1-e 0+e],c3);plot([0 1 1 0 0],[0 0 1 1 0]);
  mux : Mux  Inputs=1
      mask Display: e = 0.06;c1 = [120 150 230]/255;c2 = ([120 150 230]+0)/383;c3 = ([120 150 230]+128)/383;patch([0 1 1 0],[0 0 1 1],c1);patch([0 1 1 1-e 1-e 0+e],[0 0 1 1-e 0+e 0+e],c2);patch([0 0 1 1-e 0+e 0+e],[0 1 1 1-e 1-e 0+e],c3);plot([0 1 1 0 0],[0 0 1 1 0]);disp('Mux')
  "pd{4,3}" : Outport
      mask Display: e = 0.06;c1 = [120 230 180]/255;c2 = ([120 230 180]+0)/(256+128);c3 = ([120 230 180]+128)/(256+128);patch([0 1 1 0],[0 0 1 1],c1);patch([0 1 1 1-e 1-e 0+e],[0 0 1 1-e 0+e 0+e],c2);patch([0 0 1 1-e 0+e 0+e],[0 1 1 1-e 1-e 0+e],c3);plot([0 1 1 0 0],[0 0 1 1 0]);
  wires:
  "p{4}"/1 -> mux/1
  mux/1 -> "pd{4,3}"/1
